simulink model "Full_quadcopter_CO"  (Simulink 7.7)
settings: Solver=ode45  StartTime=0.0  StopTime=10.0  RelTol=1e-3
values from neighbouring files (symbols this model uses):
  b = 9.7575e-6    (= 9.7575e-06)    [ForcesTest.m]    (also in QuadDynamics.m = 9.937e-09; QuadDynamicsC.m = 1.7246e-06; Quadparameters.m = 3.13e-05; quadparam.m = 3.13e-05)
  g = 9.81    [ForcesTest.m]    (also in QuadDynamics.m; QuadDynamicsC.m; Quadparameters.m; quadparam.m)
  k = k+1    (= 1)    [ForcesTest.m]    (also in QuadDynamics.m = 3.82192307692e-10; QuadDynamicsC.m = 6.633e-08)
  m = 1.282    [ForcesTest.m]    (also in QuadDynamics.m = 1.284; QuadDynamicsC.m = 1.284; Quadparameters.m = 0.65; quadparam.m = 0.65)
undefined symbols (not defined in the file or in its folder): db
libraries: simulink x6
settings Model: Creator=???????  LastModifiedBy=Alexey

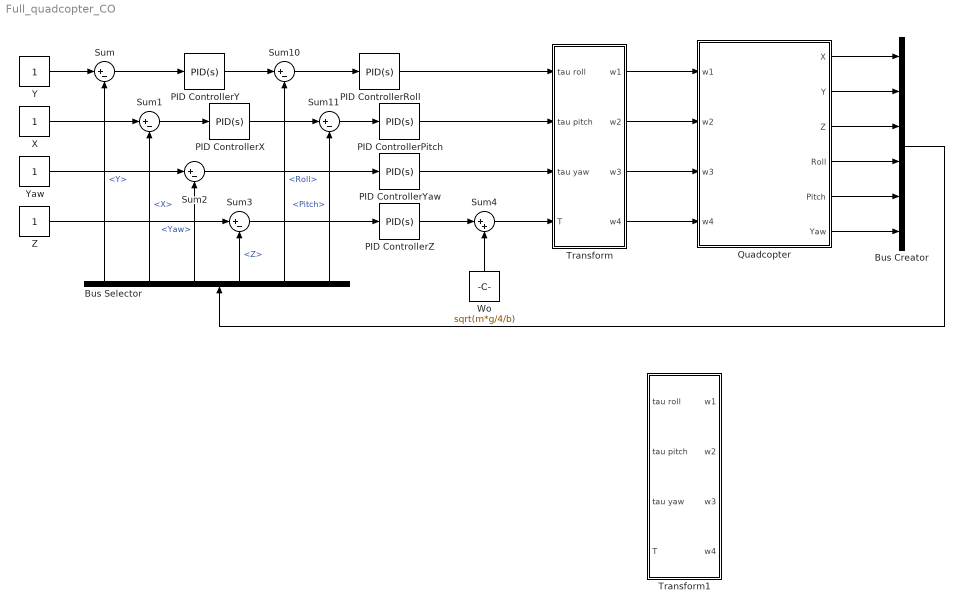
== system Full_quadcopter_CO ==
  Bus Creator : BusCreator  Inputs=6
  Bus Selector : BusSelector  OutputSignals=Y,X,Yaw,Z,Roll,Pitch
  PID ControllerPitch : simulink/Continuous/PID Controller  SystemSampleTime=-1  Controller=PID  TimeDomain=Continuous-time  SampleTime=1  IntegratorMethod=Forward Euler  FilterMethod=Forward Euler  Form=Parallel  P=1  I=1  D=0  N=100  InitialConditionSource=internal  InitialConditionForIntegrator=0  InitialConditionForFilter=0  ExternalReset=none  LimitOutput=off  UpperSaturationLimit=inf  LowerSaturationLimit=-inf  LinearizeAsGain=off  AntiWindupMode=none  Kb=1  TrackingMode=off  Kt=1  PParamMin=[]  PParamMax=[]  IParamMin=[]  IParamMax=[]  DParamMin=[]  DParamMax=[]  NParamMin=[]  NParamMax=[]  KbParamMin=[]  KbParamMax=[]  KtParamMin=[]  KtParamMax=[]  POutMin=[]  POutMax=[]  IOutMin=[]  IOutMax=[]  DOutMin=[]  DOutMax=[]  NOutMin=[]  NOutMax=[]  KbOutMin=[]  KbOutMax=[]  KtOutMin=[]  KtOutMax=[]  IntegratorOutMin=[]  IntegratorOutMax=[]  FilterOutMin=[]  FilterOutMax=[]  SumOutMin=[]  SumOutMax=[]  SumI1OutMin=[]  SumI1OutMax=[]  SumI2OutMin=[]  SumI2OutMax=[]  SumI3OutMin=[]  SumI3OutMax=[]  SumDOutMin=[]  SumDOutMax=[]  SaturationOutMin=[]  SaturationOutMax=[]  IntegratorContinuousStateAttributes=''  IntegratorStateMustResolveToSignalObject=off  IntegratorRTWStateStorageClass=Auto  FilterContinuousStateAttributes=''  FilterStateMustResolveToSignalObject=off  FilterRTWStateStorageClass=Auto
  PID ControllerRoll : simulink/Continuous/PID Controller  SystemSampleTime=-1  Controller=PID  TimeDomain=Continuous-time  SampleTime=1  IntegratorMethod=Forward Euler  FilterMethod=Forward Euler  Form=Parallel  P=1  I=1  D=0  N=100  InitialConditionSource=internal  InitialConditionForIntegrator=0  InitialConditionForFilter=0  ExternalReset=none  LimitOutput=off  UpperSaturationLimit=inf  LowerSaturationLimit=-inf  LinearizeAsGain=off  AntiWindupMode=none  Kb=1  TrackingMode=off  Kt=1  PParamMin=[]  PParamMax=[]  IParamMin=[]  IParamMax=[]  DParamMin=[]  DParamMax=[]  NParamMin=[]  NParamMax=[]  KbParamMin=[]  KbParamMax=[]  KtParamMin=[]  KtParamMax=[]  POutMin=[]  POutMax=[]  IOutMin=[]  IOutMax=[]  DOutMin=[]  DOutMax=[]  NOutMin=[]  NOutMax=[]  KbOutMin=[]  KbOutMax=[]  KtOutMin=[]  KtOutMax=[]  IntegratorOutMin=[]  IntegratorOutMax=[]  FilterOutMin=[]  FilterOutMax=[]  SumOutMin=[]  SumOutMax=[]  SumI1OutMin=[]  SumI1OutMax=[]  SumI2OutMin=[]  SumI2OutMax=[]  SumI3OutMin=[]  SumI3OutMax=[]  SumDOutMin=[]  SumDOutMax=[]  SaturationOutMin=[]  SaturationOutMax=[]  IntegratorContinuousStateAttributes=''  IntegratorStateMustResolveToSignalObject=off  IntegratorRTWStateStorageClass=Auto  FilterContinuousStateAttributes=''  FilterStateMustResolveToSignalObject=off  FilterRTWStateStorageClass=Auto
  PID ControllerX : simulink/Continuous/PID Controller  SystemSampleTime=-1  Controller=PID  TimeDomain=Continuous-time  SampleTime=1  IntegratorMethod=Forward Euler  FilterMethod=Forward Euler  Form=Parallel  P=1  I=1  D=0  N=100  InitialConditionSource=internal  InitialConditionForIntegrator=0  InitialConditionForFilter=0  ExternalReset=none  LimitOutput=off  UpperSaturationLimit=inf  LowerSaturationLimit=-inf  LinearizeAsGain=off  AntiWindupMode=none  Kb=1  TrackingMode=off  Kt=1  PParamMin=[]  PParamMax=[]  IParamMin=[]  IParamMax=[]  DParamMin=[]  DParamMax=[]  NParamMin=[]  NParamMax=[]  KbParamMin=[]  KbParamMax=[]  KtParamMin=[]  KtParamMax=[]  POutMin=[]  POutMax=[]  IOutMin=[]  IOutMax=[]  DOutMin=[]  DOutMax=[]  NOutMin=[]  NOutMax=[]  KbOutMin=[]  KbOutMax=[]  KtOutMin=[]  KtOutMax=[]  IntegratorOutMin=[]  IntegratorOutMax=[]  FilterOutMin=[]  FilterOutMax=[]  SumOutMin=[]  SumOutMax=[]  SumI1OutMin=[]  SumI1OutMax=[]  SumI2OutMin=[]  SumI2OutMax=[]  SumI3OutMin=[]  SumI3OutMax=[]  SumDOutMin=[]  SumDOutMax=[]  SaturationOutMin=[]  SaturationOutMax=[]  IntegratorContinuousStateAttributes=''  IntegratorStateMustResolveToSignalObject=off  IntegratorRTWStateStorageClass=Auto  FilterContinuousStateAttributes=''  FilterStateMustResolveToSignalObject=off  FilterRTWStateStorageClass=Auto
  PID ControllerY : simulink/Continuous/PID Controller  SystemSampleTime=-1  Controller=PID  TimeDomain=Continuous-time  SampleTime=1  IntegratorMethod=Forward Euler  FilterMethod=Forward Euler  Form=Parallel  P=1  I=1  D=0  N=100  InitialConditionSource=internal  InitialConditionForIntegrator=0  InitialConditionForFilter=0  ExternalReset=none  LimitOutput=off  UpperSaturationLimit=inf  LowerSaturationLimit=-inf  LinearizeAsGain=off  AntiWindupMode=none  Kb=1  TrackingMode=off  Kt=1  PParamMin=[]  PParamMax=[]  IParamMin=[]  IParamMax=[]  DParamMin=[]  DParamMax=[]  NParamMin=[]  NParamMax=[]  KbParamMin=[]  KbParamMax=[]  KtParamMin=[]  KtParamMax=[]  POutMin=[]  POutMax=[]  IOutMin=[]  IOutMax=[]  DOutMin=[]  DOutMax=[]  NOutMin=[]  NOutMax=[]  KbOutMin=[]  KbOutMax=[]  KtOutMin=[]  KtOutMax=[]  IntegratorOutMin=[]  IntegratorOutMax=[]  FilterOutMin=[]  FilterOutMax=[]  SumOutMin=[]  SumOutMax=[]  SumI1OutMin=[]  SumI1OutMax=[]  SumI2OutMin=[]  SumI2OutMax=[]  SumI3OutMin=[]  SumI3OutMax=[]  SumDOutMin=[]  SumDOutMax=[]  SaturationOutMin=[]  SaturationOutMax=[]  IntegratorContinuousStateAttributes=''  IntegratorStateMustResolveToSignalObject=off  IntegratorRTWStateStorageClass=Auto  FilterContinuousStateAttributes=''  FilterStateMustResolveToSignalObject=off  FilterRTWStateStorageClass=Auto
  PID ControllerYaw : simulink/Continuous/PID Controller  SystemSampleTime=-1  Controller=PID  TimeDomain=Continuous-time  SampleTime=1  IntegratorMethod=Forward Euler  FilterMethod=Forward Euler  Form=Parallel  P=1  I=1  D=0  N=100  InitialConditionSource=internal  InitialConditionForIntegrator=0  InitialConditionForFilter=0  ExternalReset=none  LimitOutput=off  UpperSaturationLimit=inf  LowerSaturationLimit=-inf  LinearizeAsGain=off  AntiWindupMode=none  Kb=1  TrackingMode=off  Kt=1  PParamMin=[]  PParamMax=[]  IParamMin=[]  IParamMax=[]  DParamMin=[]  DParamMax=[]  NParamMin=[]  NParamMax=[]  KbParamMin=[]  KbParamMax=[]  KtParamMin=[]  KtParamMax=[]  POutMin=[]  POutMax=[]  IOutMin=[]  IOutMax=[]  DOutMin=[]  DOutMax=[]  NOutMin=[]  NOutMax=[]  KbOutMin=[]  KbOutMax=[]  KtOutMin=[]  KtOutMax=[]  IntegratorOutMin=[]  IntegratorOutMax=[]  FilterOutMin=[]  FilterOutMax=[]  SumOutMin=[]  SumOutMax=[]  SumI1OutMin=[]  SumI1OutMax=[]  SumI2OutMin=[]  SumI2OutMax=[]  SumI3OutMin=[]  SumI3OutMax=[]  SumDOutMin=[]  SumDOutMax=[]  SaturationOutMin=[]  SaturationOutMax=[]  IntegratorContinuousStateAttributes=''  IntegratorStateMustResolveToSignalObject=off  IntegratorRTWStateStorageClass=Auto  FilterContinuousStateAttributes=''  FilterStateMustResolveToSignalObject=off  FilterRTWStateStorageClass=Auto
  PID ControllerZ : simulink/Continuous/PID Controller  SystemSampleTime=-1  Controller=PID  TimeDomain=Continuous-time  SampleTime=1  IntegratorMethod=Forward Euler  FilterMethod=Forward Euler  Form=Parallel  P=1  I=1  D=0  N=100  InitialConditionSource=internal  InitialConditionForIntegrator=0  InitialConditionForFilter=0  ExternalReset=none  LimitOutput=off  UpperSaturationLimit=inf  LowerSaturationLimit=-inf  LinearizeAsGain=off  AntiWindupMode=none  Kb=1  TrackingMode=off  Kt=1  PParamMin=[]  PParamMax=[]  IParamMin=[]  IParamMax=[]  DParamMin=[]  DParamMax=[]  NParamMin=[]  NParamMax=[]  KbParamMin=[]  KbParamMax=[]  KtParamMin=[]  KtParamMax=[]  POutMin=[]  POutMax=[]  IOutMin=[]  IOutMax=[]  DOutMin=[]  DOutMax=[]  NOutMin=[]  NOutMax=[]  KbOutMin=[]  KbOutMax=[]  KtOutMin=[]  KtOutMax=[]  IntegratorOutMin=[]  IntegratorOutMax=[]  FilterOutMin=[]  FilterOutMax=[]  SumOutMin=[]  SumOutMax=[]  SumI1OutMin=[]  SumI1OutMax=[]  SumI2OutMin=[]  SumI2OutMax=[]  SumI3OutMin=[]  SumI3OutMax=[]  SumDOutMin=[]  SumDOutMax=[]  SaturationOutMin=[]  SaturationOutMax=[]  IntegratorContinuousStateAttributes=''  IntegratorStateMustResolveToSignalObject=off  IntegratorRTWStateStorageClass=Auto  FilterContinuousStateAttributes=''  FilterStateMustResolveToSignalObject=off  FilterRTWStateStorageClass=Auto
  Quadcopter : Subsystem
  Sum{,1..3,10..11} (6 alike) : Sum  Inputs=|+-
  Sum4 : Sum  Inputs=|++
  Transform : Subsystem
  Transform1 : Subsystem
  Wo : Constant  Value=sqrt(m*g/4/b)
  X : Constant
  Y : Constant
  Yaw : Constant
  Z : Constant
  wires:
  Y/1 -> Sum/1
  X/1 -> Sum1/1
  Yaw/1 -> Sum2/1
  Z/1 -> Sum3/1
  Sum/1 -> PID ControllerY/1
  Sum1/1 -> PID ControllerX/1
  Sum2/1 -> PID ControllerYaw/1
  Sum3/1 -> PID ControllerZ/1
  Transform/1(w1) -> Quadcopter/1(w1)
  Transform/2(w2) -> Quadcopter/2(w2)
  Transform/3(w3) -> Quadcopter/3(w3)
  Transform/4(w4) -> Quadcopter/4(w4)
  PID ControllerYaw/1 -> Transform/3(tau yaw)
  Sum4/1 -> Transform/4(T)
  PID ControllerZ/1 -> Sum4/1
  Wo/1 -> Sum4/2
  Bus Selector/1 -> Sum/2  "<Y>"
  Bus Selector/2 -> Sum1/2  "<X>"
  Bus Selector/3 -> Sum2/2  "<Yaw>"
  Bus Selector/4 -> Sum3/2  "<Z>"
  Bus Creator/1 -> Bus Selector/1
  Quadcopter/1(X) -> Bus Creator/1
  Quadcopter/2(Y) -> Bus Creator/2
  Quadcopter/3(Z) -> Bus Creator/3
  Quadcopter/4(Roll) -> Bus Creator/4
  Quadcopter/5(Pitch) -> Bus Creator/5
  Quadcopter/6(Yaw) -> Bus Creator/6
  PID ControllerY/1 -> Sum10/1
  PID ControllerX/1 -> Sum11/1
  Bus Selector/6 -> Sum11/2  "<Pitch>"
  Sum11/1 -> PID ControllerPitch/1
  PID ControllerPitch/1 -> Transform/2(tau pitch)
  Sum10/1 -> PID ControllerRoll/1
  PID ControllerRoll/1 -> Transform/1(tau roll)
  Bus Selector/5 -> Sum10/2  "<Roll>"

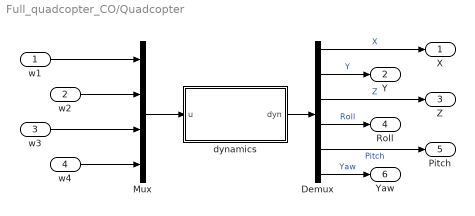
== system Full_quadcopter_CO/Quadcopter ==
  w1 : Inport
  w2 : Inport  Port=2
  w3 : Inport  Port=3
  w4 : Inport  Port=4
  Demux : Demux  Outputs=6
  Mux : Mux
  dynamics : Stateflow chart  TreatAsAtomicUnit=on
  X : Outport
  Y : Outport  Port=2
  Z : Outport  Port=3
  Roll : Outport  Port=4
  Pitch : Outport  Port=5
  Yaw : Outport  Port=6
  wires:
  w1/1 -> Mux/1
  w2/1 -> Mux/2
  w3/1 -> Mux/3
  w4/1 -> Mux/4
  Demux/1 -> X/1  "X"
  Demux/2 -> Y/1  "Y"
  Demux/3 -> Z/1  "Z"
  Demux/4 -> Roll/1  "Roll"
  Demux/5 -> Pitch/1  "Pitch"
  Demux/6 -> Yaw/1  "Yaw"
  Mux/1 -> dynamics/1(u)
  dynamics/1(dyn) -> Demux/1

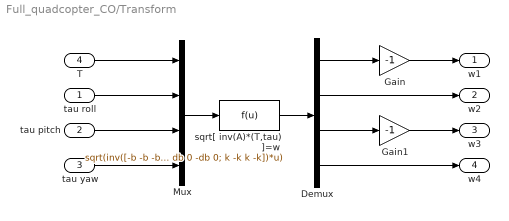
== system Full_quadcopter_CO/Transform ==
  tau roll : Inport
  tau pitch : Inport  Port=2
  tau yaw : Inport  Port=3
  T : Inport  Port=4
  Demux : Demux
  Gain : Gain  Gain=-1
  Gain1 : Gain  Gain=-1
  Mux : Mux
  sqrt[ inv(A)*(T,tau) ]=w : Fcn  Expr=sqrt(inv([-b -b -b -b; 0 -db 0 db; db 0 -db 0; k -k k -k])*u)
  w1 : Outport
  w2 : Outport  Port=2
  w3 : Outport  Port=3
  w4 : Outport  Port=4
  wires:
  Gain1/1 -> w3/1
  Gain/1 -> w1/1
  tau yaw/1 -> Mux/4
  tau pitch/1 -> Mux/3
  tau roll/1 -> Mux/2
  T/1 -> Mux/1
  Demux/4 -> w4/1
  Demux/3 -> Gain1/1
  Demux/2 -> w2/1
  Demux/1 -> Gain/1
  Mux/1 -> sqrt[ inv(A)*(T,tau) ]=w/1
  sqrt[ inv(A)*(T,tau) ]=w/1 -> Demux/1

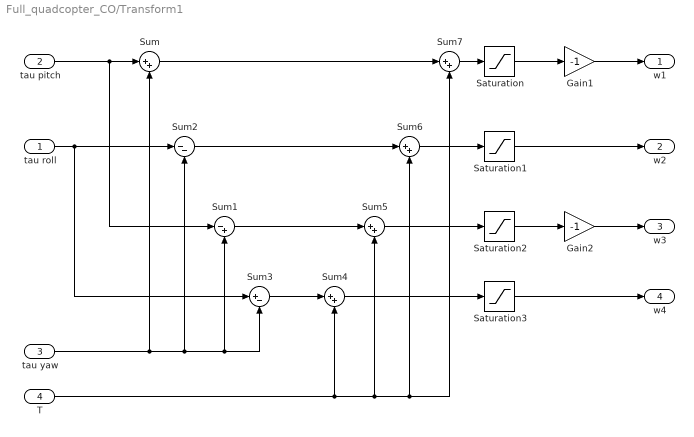
== system Full_quadcopter_CO/Transform1 ==
  tau roll : Inport
  tau pitch : Inport  Port=2
  tau yaw : Inport  Port=3
  T : Inport  Port=4
  Gain1 : Gain  Gain=-1
  Gain2 : Gain  Gain=-1
  Saturation{,1..3} (4 alike) : Saturate
  Sum{,4..7} (5 alike) : Sum  Inputs=|++
  Sum1 : Sum  Inputs=|-+
  Sum2 : Sum  Inputs=|--
  Sum3 : Sum  Inputs=|+-
  w1 : Outport
  w2 : Outport  Port=2
  w3 : Outport  Port=3
  w4 : Outport  Port=4
  wires:
  tau pitch/1 -> Sum/1, Sum1/1
  tau roll/1 -> Sum3/1, Sum2/1
  tau yaw/1 -> Sum/2, Sum2/2, Sum1/2, Sum3/2
  Sum3/1 -> Sum4/1
  Sum1/1 -> Sum5/1
  Sum2/1 -> Sum6/1
  Sum/1 -> Sum7/1
  T/1 -> Sum4/2, Sum5/2, Sum6/2, Sum7/2
  Sum7/1 -> Saturation/1
  Sum6/1 -> Saturation1/1
  Sum5/1 -> Saturation2/1
  Sum4/1 -> Saturation3/1
  Saturation/1 -> Gain1/1
  Saturation1/1 -> w2/1
  Saturation2/1 -> Gain2/1
  Saturation3/1 -> w4/1
  Gain1/1 -> w1/1
  Gain2/1 -> w3/1

== matlab function Quadcopter/dynamics ==
  data: u input double; dyn output double
function dyn = quad_dynamics(u)
w = u(1:4);

l=0.3;
b=0.001;
k=0.001;
m=1;
g=9.81;

Ixx = 0;
Iyy = 0;
Izz = 0;
J = diag([Ixx Iyy Izz]);

D(:,1) = [l;0;h];
D(:,2) = [0;l;h];
D(:,3) = [-l;0;h];
D(:,4) = [0;-l;h];

R = [cos(Theta)*cos(Phi)          sin(Psi)*sin(Theta)*cos(Phi)-cos(Psi)*sin(Phi)          cos(Psi)*sin(Theta)*cos(Phi)+sin(Psi)*sin(Phi);
         cos(Theta)*sin(Phi)            sin(Psi)*sin(Theta)*sin(Phi)+cos(Psi)*cos(Phi)         cos(Psi)*sin(Theta)*sin(Phi)-sin(Psi)*cos(Phi);
         -sin(Theta)                           sin(Psi)*cos(Theta)                                                       cos(Psi)*cos(Theta)];

Rr = (1/cos(Theta)) * [0                      sin(Psi)                            cos(Psi);             
                                                            0                      cos(Psi)*cos(Theta)       -sin(Psi)*cos(Theta);
                                                            cos(Theta)      sin(Psi)*sin(Theta)          cos(Psi)*sin(Theta)];

for i=1:4
 T(i) = b * w(i)^2 * [0;0;1];  
 Q(i) = k * w(i)^2 * [0;0;1];    
 tau(i) = cross(T(i),D(i));   
end

dXYZ = Velocity;
dTheta = Rr*Omega;

dVelocity = g * [0;0;1] + R * (1 / m) * T(i);
dOmega = (cross(-Omega,J*Omega) + tau(i)) / J; 

dyn = [dXYZ; dTheta; dVelocity; dOmega];   
end
